simulink model "simulationBallCatching"  (R2017b)
settings: Solver=VariableStepAuto  StartTime=0.0  StopTime=simTime  MaxStep=0.001  RelTol=1e-3  EnableMultiTasking=on
undefined symbols (not defined in the file or in its folder): ball_radius, basket_side, contact_damping, contact_stiffness, dt, g, I11, I22, I33, Kd_phi, Kd_psi, Kd_theta, Kd_x, Kd_y, Kd_z, Kp_phi, Kp_psi, Kp_theta, Kp_x, Kp_y, Kp_z, m, m_ball, T, X, Y, Z, z0
libraries: nesl_utility x86, sm_lib x74, Contact_Forces_Lib x20, simulink x10
(part 3 of 4)

== system simulationBallCatching/Plant/Basket/Contact2 ==
  Bus Creator : BusCreator  Inputs=3
  Check Sphere on Plane : Subsystem
  Demux : Subsystem
  Enable Outputs : Subsystem
  External Force and Torque PlaB : sm_lib/Forces and Torques/External Force and Torque  ForceResolutionFrame=AttachedFrame  EnableForceX=off  EnableForceY=off  EnableForceZ=off  EnableForce=on  TorqueResolutionFrame=AttachedFrame  EnableTorqueX=off  EnableTorqueY=off  EnableTorqueZ=off  EnableTorque=on
  External Force and Torque SphF : sm_lib/Forces and Torques/External Force and Torque  ForceResolutionFrame=AttachedFrame  EnableForceX=off  EnableForceY=off  EnableForceZ=off  EnableForce=on  TorqueResolutionFrame=AttachedFrame  EnableTorqueX=off  EnableTorqueY=off  EnableTorqueZ=off  EnableTorque=on
  Forces : Subsystem
  If1 : If  IfExpression=u1>0
  Merge : Merge
  No Force : Subsystem  TreatAsAtomicUnit=on
  Sensing : Subsystem
  Transform nZ : sm_lib/Frames and Transforms/Rigid Transform  TranslationMethod=StandardAxis  TranslationStandardOffset=plane_depth-vis_len_plaBz/2  TranslationLengthUnit=m  TranslationStandardAxis=-Z  TranslationCartesianOffset=[0 0 0]  TranslationROffset=0  TranslationROffsetUnits=m  TranslationZOffset=0  TranslationZOffsetUnits=m  TranslationThetaOffset=0  TranslationThetaOffsetUnits=deg  RotationMethod=None  RotationAngleUnits=deg  RotationStandardAxis=+Z  RotationAngle=0.0  RotationArbitraryAxis=[0 0 1]  FollAlignAxisA=+X  BaseAlignAxisA=+Y  FollAlignAxisB=+Y  BaseAlignAxisB=+Z  RotationSequenceAxes=FollowerAxes  RotationSequence=XYX  RotationSequenceAngles=[0 0 0]  RotationSequenceAnglesUnits=deg  RotationMatrix=[1 0 0; 0 1 0; 0 0 1]
  Transform pZ : sm_lib/Frames and Transforms/Rigid Transform  TranslationMethod=StandardAxis  TranslationStandardOffset=plane_depth-vis_len_plaBz/2  TranslationLengthUnit=m  TranslationStandardAxis=+Z  TranslationCartesianOffset=[0 0 0]  TranslationROffset=0  TranslationROffsetUnits=m  TranslationZOffset=0  TranslationZOffsetUnits=m  TranslationThetaOffset=0  TranslationThetaOffsetUnits=deg  RotationMethod=None  RotationAngleUnits=deg  RotationStandardAxis=+Z  RotationAngle=0.0  RotationArbitraryAxis=[0 0 1]  FollAlignAxisA=+X  BaseAlignAxisA=+Y  FollAlignAxisB=+Y  BaseAlignAxisB=+Z  RotationSequenceAxes=FollowerAxes  RotationSequence=XYX  RotationSequenceAngles=[0 0 0]  RotationSequenceAnglesUnits=deg  RotationMatrix=[1 0 0; 0 1 0; 0 0 1]
  Visual CirF : sm_lib/Body Elements/Solid  InertiaType=CalculateFromGeometry  Mass=1  MassUnits=kg  CenterOfMass=[0 0 0]  CenterOfMassUnits=m  MomentsOfInertia=[1 1 1]  MomentsOfInertiaUnits=kg*m^2  ProductsOfInertia=[0 0 0]  ProductsOfInertiaUnits=kg*m^2  DensityBased=on  Density=0  DensityUnits=kg/(m^3)  DoExposeReferenceFrame=on  SerializedFrames=<Frames/>  GraphicType=FromGeometry  MarkerShape=Sphere  MarkerSize=10  GraphicVisPropType=SimpleVisualProperties  GraphicDiffuseColor=vis_clr  GraphicSpecularColor=[0.5 0.5 0.5 1.0]  GraphicAmbientColor=[0.15 0.15 0.15 1.0]  GraphicEmissiveColor=[0.0 0.0 0.0 1.0]  GraphicShininess=75  GraphicOpacity=vis_opc*vis_opc_en  GeometryShape=Sphere  RectangleSize=[1 1]  RectangleSizeUnits=m  BrickDimensions=[1 1 1]  BrickDimensionUnits=m  CylinderRadius=1  CylinderRadiusUnits=m  CylinderLength=1  CylinderLengthUnits=m  SphereRadius=sphere_rad  SphereRadiusUnits=m  EllipsoidRadii=[1 1 1]  EllipsoidRadiiUnits=m  ExtrusionCrossSection=[1 1; -1 1; -1 -1; 1 -1]  ExtrusionCrossSectionUnits=m  ExtrusionLength=1  ExtrusionLengthUnits=m  PolygonNumSides=3  PolygonOuterRadius=1  PolygonOuterRadiusUnits=m  ExtGeomFileType=STEP  ExtGeomFileUnits=m  RevolutionCrossSection=[1 1; 1 -1; 2 -1; 2 1]  RevolutionCrossSectionUnits=m  RevolutionExtent=Full  RevolutionAngle=180  RevolutionAngleUnits=deg
  Visual PlaBnZ : sm_lib/Body Elements/Solid  InertiaType=CalculateFromGeometry  Mass=1  MassUnits=kg  CenterOfMass=[0 0 0]  CenterOfMassUnits=m  MomentsOfInertia=[1 1 1]  MomentsOfInertiaUnits=kg*m^2  ProductsOfInertia=[0 0 0]  ProductsOfInertiaUnits=kg*m^2  DensityBased=on  Density=0  DensityUnits=kg/(m^3)  DoExposeReferenceFrame=on  SerializedFrames=<Frames/>  GraphicType=FromGeometry  MarkerShape=Sphere  MarkerSize=10  GraphicVisPropType=SimpleVisualProperties  GraphicDiffuseColor=vis_clr  GraphicSpecularColor=[0.5 0.5 0.5 1.0]  GraphicAmbientColor=[0.15 0.15 0.15 1.0]  GraphicEmissiveColor=[0.0 0.0 0.0 1.0]  GraphicShininess=75  GraphicOpacity=vis_opc*vis_opc_en  GeometryShape=Brick  RectangleSize=[1 1]  RectangleSizeUnits=m  BrickDimensions=[plane_lenx plane_leny vis_len_plaBz]  BrickDimensionUnits=m  CylinderRadius=1  CylinderRadiusUnits=m  CylinderLength=1  CylinderLengthUnits=m  SphereRadius=1  SphereRadiusUnits=m  EllipsoidRadii=[1 1 1]  EllipsoidRadiiUnits=m  ExtrusionCrossSection=[1 1; -1 1; -1 -1; 1 -1]  ExtrusionCrossSectionUnits=m  ExtrusionLength=1  ExtrusionLengthUnits=m  PolygonNumSides=3  PolygonOuterRadius=1  PolygonOuterRadiusUnits=m  ExtGeomFileType=STEP  ExtGeomFileUnits=m  RevolutionCrossSection=[1 1; 1 -1; 2 -1; 2 1]  RevolutionCrossSectionUnits=m  RevolutionExtent=Full  RevolutionAngle=180  RevolutionAngleUnits=deg
  Visual PlaBpZ : sm_lib/Body Elements/Solid  InertiaType=CalculateFromGeometry  Mass=1  MassUnits=kg  CenterOfMass=[0 0 0]  CenterOfMassUnits=m  MomentsOfInertia=[1 1 1]  MomentsOfInertiaUnits=kg*m^2  ProductsOfInertia=[0 0 0]  ProductsOfInertiaUnits=kg*m^2  DensityBased=on  Density=0  DensityUnits=kg/(m^3)  DoExposeReferenceFrame=on  SerializedFrames=<Frames/>  GraphicType=FromGeometry  MarkerShape=Sphere  MarkerSize=10  GraphicVisPropType=SimpleVisualProperties  GraphicDiffuseColor=vis_clr  GraphicSpecularColor=[0.5 0.5 0.5 1.0]  GraphicAmbientColor=[0.15 0.15 0.15 1.0]  GraphicEmissiveColor=[0.0 0.0 0.0 1.0]  GraphicShininess=75  GraphicOpacity=vis_opc*vis_opc_en  GeometryShape=Brick  RectangleSize=[1 1]  RectangleSizeUnits=m  BrickDimensions=[plane_lenx plane_leny vis_len_plaBz]  BrickDimensionUnits=m  CylinderRadius=1  CylinderRadiusUnits=m  CylinderLength=1  CylinderLengthUnits=m  SphereRadius=1  SphereRadiusUnits=m  EllipsoidRadii=[1 1 1]  EllipsoidRadiiUnits=m  ExtrusionCrossSection=[1 1; -1 1; -1 -1; 1 -1]  ExtrusionCrossSectionUnits=m  ExtrusionLength=1  ExtrusionLengthUnits=m  PolygonNumSides=3  PolygonOuterRadius=1  PolygonOuterRadiusUnits=m  ExtGeomFileType=STEP  ExtGeomFileUnits=m  RevolutionCrossSection=[1 1; 1 -1; 2 -1; 2 1]  RevolutionCrossSectionUnits=m  RevolutionExtent=Full  RevolutionAngle=180  RevolutionAngleUnits=deg
  SphF : PMIOPort  Port=1  Side=Left
  PlaB : PMIOPort  Port=2  Side=Right
  Out : Outport
  wires:
  Check Sphere on Plane/1(En) -> If1/1, Enable Outputs/2(En)
  Enable Outputs/1(Out) -> Out/1
  Bus Creator/1 -> Enable Outputs/3(FrameSep)  "Frame Sep"
  Forces/2(Out) -> Enable Outputs/1(Frc)
  Merge/1 -> Demux/1(Frc)  "FSph"
  Forces/1(Frc) -> Merge/2
  Sensing/4(vz) -> Forces/4(vz)
  Sensing/5(R) -> Forces/5(R)
  Sensing/3(z) -> Forces/3(z), Bus Creator/3  "z"
  Sensing/6(wx) -> Forces/6(wx)
  Sensing/7(wy) -> Forces/7(wy)
  Sensing/8(vx) -> Forces/8(vx)
  Sensing/9(vy) -> Forces/9(vy)
  Sensing/1(x) -> Forces/1(x), Bus Creator/1, Check Sphere on Plane/1(x)  "x"
  Sensing/2(y) -> Forces/2(y), Bus Creator/2, Check Sphere on Plane/2(y)  "y"
  If1/1 -> Forces/Action
  If1/2 -> No Force/Action
  No Force/1(Frc) -> Merge/1
  connections:
  SphF/RConn1 -- Sensing/LConn1 -- Visual CirF/RConn1 -- External Force and Torque SphF/RConn1
  PlaB/RConn1 -- Sensing/LConn2 -- External Force and Torque PlaB/RConn1 -- Transform pZ/LConn1 -- Transform nZ/LConn1
  Demux/RConn1 -- External Force and Torque SphF/LConn1
  Demux/RConn2 -- External Force and Torque SphF/LConn2
  Demux/RConn3 -- External Force and Torque PlaB/LConn1
  Demux/RConn4 -- External Force and Torque PlaB/LConn2
  Transform pZ/RConn1 -- Visual PlaBpZ/RConn1
  Transform nZ/RConn1 -- Visual PlaBnZ/RConn1

== system simulationBallCatching/Plant/Basket/Contact3 ==
  Bus Creator : BusCreator  Inputs=3
  Check Sphere on Plane : Subsystem
  Demux : Subsystem
  Enable Outputs : Subsystem
  External Force and Torque PlaB : sm_lib/Forces and Torques/External Force and Torque  ForceResolutionFrame=AttachedFrame  EnableForceX=off  EnableForceY=off  EnableForceZ=off  EnableForce=on  TorqueResolutionFrame=AttachedFrame  EnableTorqueX=off  EnableTorqueY=off  EnableTorqueZ=off  EnableTorque=on
  External Force and Torque SphF : sm_lib/Forces and Torques/External Force and Torque  ForceResolutionFrame=AttachedFrame  EnableForceX=off  EnableForceY=off  EnableForceZ=off  EnableForce=on  TorqueResolutionFrame=AttachedFrame  EnableTorqueX=off  EnableTorqueY=off  EnableTorqueZ=off  EnableTorque=on
  Forces : Subsystem
  If1 : If  IfExpression=u1>0
  Merge : Merge
  No Force : Subsystem  TreatAsAtomicUnit=on
  Sensing : Subsystem
  Transform nZ : sm_lib/Frames and Transforms/Rigid Transform  TranslationMethod=StandardAxis  TranslationStandardOffset=plane_depth-vis_len_plaBz/2  TranslationLengthUnit=m  TranslationStandardAxis=-Z  TranslationCartesianOffset=[0 0 0]  TranslationROffset=0  TranslationROffsetUnits=m  TranslationZOffset=0  TranslationZOffsetUnits=m  TranslationThetaOffset=0  TranslationThetaOffsetUnits=deg  RotationMethod=None  RotationAngleUnits=deg  RotationStandardAxis=+Z  RotationAngle=0.0  RotationArbitraryAxis=[0 0 1]  FollAlignAxisA=+X  BaseAlignAxisA=+Y  FollAlignAxisB=+Y  BaseAlignAxisB=+Z  RotationSequenceAxes=FollowerAxes  RotationSequence=XYX  RotationSequenceAngles=[0 0 0]  RotationSequenceAnglesUnits=deg  RotationMatrix=[1 0 0; 0 1 0; 0 0 1]
  Transform pZ : sm_lib/Frames and Transforms/Rigid Transform  TranslationMethod=StandardAxis  TranslationStandardOffset=plane_depth-vis_len_plaBz/2  TranslationLengthUnit=m  TranslationStandardAxis=+Z  TranslationCartesianOffset=[0 0 0]  TranslationROffset=0  TranslationROffsetUnits=m  TranslationZOffset=0  TranslationZOffsetUnits=m  TranslationThetaOffset=0  TranslationThetaOffsetUnits=deg  RotationMethod=None  RotationAngleUnits=deg  RotationStandardAxis=+Z  RotationAngle=0.0  RotationArbitraryAxis=[0 0 1]  FollAlignAxisA=+X  BaseAlignAxisA=+Y  FollAlignAxisB=+Y  BaseAlignAxisB=+Z  RotationSequenceAxes=FollowerAxes  RotationSequence=XYX  RotationSequenceAngles=[0 0 0]  RotationSequenceAnglesUnits=deg  RotationMatrix=[1 0 0; 0 1 0; 0 0 1]
  Visual CirF : sm_lib/Body Elements/Solid  InertiaType=CalculateFromGeometry  Mass=1  MassUnits=kg  CenterOfMass=[0 0 0]  CenterOfMassUnits=m  MomentsOfInertia=[1 1 1]  MomentsOfInertiaUnits=kg*m^2  ProductsOfInertia=[0 0 0]  ProductsOfInertiaUnits=kg*m^2  DensityBased=on  Density=0  DensityUnits=kg/(m^3)  DoExposeReferenceFrame=on  SerializedFrames=<Frames/>  GraphicType=FromGeometry  MarkerShape=Sphere  MarkerSize=10  GraphicVisPropType=SimpleVisualProperties  GraphicDiffuseColor=vis_clr  GraphicSpecularColor=[0.5 0.5 0.5 1.0]  GraphicAmbientColor=[0.15 0.15 0.15 1.0]  GraphicEmissiveColor=[0.0 0.0 0.0 1.0]  GraphicShininess=75  GraphicOpacity=vis_opc*vis_opc_en  GeometryShape=Sphere  RectangleSize=[1 1]  RectangleSizeUnits=m  BrickDimensions=[1 1 1]  BrickDimensionUnits=m  CylinderRadius=1  CylinderRadiusUnits=m  CylinderLength=1  CylinderLengthUnits=m  SphereRadius=sphere_rad  SphereRadiusUnits=m  EllipsoidRadii=[1 1 1]  EllipsoidRadiiUnits=m  ExtrusionCrossSection=[1 1; -1 1; -1 -1; 1 -1]  ExtrusionCrossSectionUnits=m  ExtrusionLength=1  ExtrusionLengthUnits=m  PolygonNumSides=3  PolygonOuterRadius=1  PolygonOuterRadiusUnits=m  ExtGeomFileType=STEP  ExtGeomFileUnits=m  RevolutionCrossSection=[1 1; 1 -1; 2 -1; 2 1]  RevolutionCrossSectionUnits=m  RevolutionExtent=Full  RevolutionAngle=180  RevolutionAngleUnits=deg
  Visual PlaBnZ : sm_lib/Body Elements/Solid  InertiaType=CalculateFromGeometry  Mass=1  MassUnits=kg  CenterOfMass=[0 0 0]  CenterOfMassUnits=m  MomentsOfInertia=[1 1 1]  MomentsOfInertiaUnits=kg*m^2  ProductsOfInertia=[0 0 0]  ProductsOfInertiaUnits=kg*m^2  DensityBased=on  Density=0  DensityUnits=kg/(m^3)  DoExposeReferenceFrame=on  SerializedFrames=<Frames/>  GraphicType=FromGeometry  MarkerShape=Sphere  MarkerSize=10  GraphicVisPropType=SimpleVisualProperties  GraphicDiffuseColor=vis_clr  GraphicSpecularColor=[0.5 0.5 0.5 1.0]  GraphicAmbientColor=[0.15 0.15 0.15 1.0]  GraphicEmissiveColor=[0.0 0.0 0.0 1.0]  GraphicShininess=75  GraphicOpacity=vis_opc*vis_opc_en  GeometryShape=Brick  RectangleSize=[1 1]  RectangleSizeUnits=m  BrickDimensions=[plane_lenx plane_leny vis_len_plaBz]  BrickDimensionUnits=m  CylinderRadius=1  CylinderRadiusUnits=m  CylinderLength=1  CylinderLengthUnits=m  SphereRadius=1  SphereRadiusUnits=m  EllipsoidRadii=[1 1 1]  EllipsoidRadiiUnits=m  ExtrusionCrossSection=[1 1; -1 1; -1 -1; 1 -1]  ExtrusionCrossSectionUnits=m  ExtrusionLength=1  ExtrusionLengthUnits=m  PolygonNumSides=3  PolygonOuterRadius=1  PolygonOuterRadiusUnits=m  ExtGeomFileType=STEP  ExtGeomFileUnits=m  RevolutionCrossSection=[1 1; 1 -1; 2 -1; 2 1]  RevolutionCrossSectionUnits=m  RevolutionExtent=Full  RevolutionAngle=180  RevolutionAngleUnits=deg
  Visual PlaBpZ : sm_lib/Body Elements/Solid  InertiaType=CalculateFromGeometry  Mass=1  MassUnits=kg  CenterOfMass=[0 0 0]  CenterOfMassUnits=m  MomentsOfInertia=[1 1 1]  MomentsOfInertiaUnits=kg*m^2  ProductsOfInertia=[0 0 0]  ProductsOfInertiaUnits=kg*m^2  DensityBased=on  Density=0  DensityUnits=kg/(m^3)  DoExposeReferenceFrame=on  SerializedFrames=<Frames/>  GraphicType=FromGeometry  MarkerShape=Sphere  MarkerSize=10  GraphicVisPropType=SimpleVisualProperties  GraphicDiffuseColor=vis_clr  GraphicSpecularColor=[0.5 0.5 0.5 1.0]  GraphicAmbientColor=[0.15 0.15 0.15 1.0]  GraphicEmissiveColor=[0.0 0.0 0.0 1.0]  GraphicShininess=75  GraphicOpacity=vis_opc*vis_opc_en  GeometryShape=Brick  RectangleSize=[1 1]  RectangleSizeUnits=m  BrickDimensions=[plane_lenx plane_leny vis_len_plaBz]  BrickDimensionUnits=m  CylinderRadius=1  CylinderRadiusUnits=m  CylinderLength=1  CylinderLengthUnits=m  SphereRadius=1  SphereRadiusUnits=m  EllipsoidRadii=[1 1 1]  EllipsoidRadiiUnits=m  ExtrusionCrossSection=[1 1; -1 1; -1 -1; 1 -1]  ExtrusionCrossSectionUnits=m  ExtrusionLength=1  ExtrusionLengthUnits=m  PolygonNumSides=3  PolygonOuterRadius=1  PolygonOuterRadiusUnits=m  ExtGeomFileType=STEP  ExtGeomFileUnits=m  RevolutionCrossSection=[1 1; 1 -1; 2 -1; 2 1]  RevolutionCrossSectionUnits=m  RevolutionExtent=Full  RevolutionAngle=180  RevolutionAngleUnits=deg
  SphF : PMIOPort  Port=1  Side=Left
  PlaB : PMIOPort  Port=2  Side=Right
  Out : Outport
  wires:
  Check Sphere on Plane/1(En) -> If1/1, Enable Outputs/2(En)
  Enable Outputs/1(Out) -> Out/1
  Bus Creator/1 -> Enable Outputs/3(FrameSep)  "Frame Sep"
  Forces/2(Out) -> Enable Outputs/1(Frc)
  Merge/1 -> Demux/1(Frc)  "FSph"
  Forces/1(Frc) -> Merge/2
  Sensing/4(vz) -> Forces/4(vz)
  Sensing/5(R) -> Forces/5(R)
  Sensing/3(z) -> Forces/3(z), Bus Creator/3  "z"
  Sensing/6(wx) -> Forces/6(wx)
  Sensing/7(wy) -> Forces/7(wy)
  Sensing/8(vx) -> Forces/8(vx)
  Sensing/9(vy) -> Forces/9(vy)
  Sensing/1(x) -> Forces/1(x), Bus Creator/1, Check Sphere on Plane/1(x)  "x"
  Sensing/2(y) -> Forces/2(y), Bus Creator/2, Check Sphere on Plane/2(y)  "y"
  If1/1 -> Forces/Action
  If1/2 -> No Force/Action
  No Force/1(Frc) -> Merge/1
  connections:
  SphF/RConn1 -- Sensing/LConn1 -- Visual CirF/RConn1 -- External Force and Torque SphF/RConn1
  PlaB/RConn1 -- Sensing/LConn2 -- External Force and Torque PlaB/RConn1 -- Transform pZ/LConn1 -- Transform nZ/LConn1
  Demux/RConn1 -- External Force and Torque SphF/LConn1
  Demux/RConn2 -- External Force and Torque SphF/LConn2
  Demux/RConn3 -- External Force and Torque PlaB/LConn1
  Demux/RConn4 -- External Force and Torque PlaB/LConn2
  Transform pZ/RConn1 -- Visual PlaBpZ/RConn1
  Transform nZ/RConn1 -- Visual PlaBnZ/RConn1

== system simulationBallCatching/Plant/Basket/Contact4 ==
  Bus Creator : BusCreator  Inputs=3
  Check Sphere on Plane : Subsystem
  Demux : Subsystem
  Enable Outputs : Subsystem
  External Force and Torque PlaB : sm_lib/Forces and Torques/External Force and Torque  ForceResolutionFrame=AttachedFrame  EnableForceX=off  EnableForceY=off  EnableForceZ=off  EnableForce=on  TorqueResolutionFrame=AttachedFrame  EnableTorqueX=off  EnableTorqueY=off  EnableTorqueZ=off  EnableTorque=on
  External Force and Torque SphF : sm_lib/Forces and Torques/External Force and Torque  ForceResolutionFrame=AttachedFrame  EnableForceX=off  EnableForceY=off  EnableForceZ=off  EnableForce=on  TorqueResolutionFrame=AttachedFrame  EnableTorqueX=off  EnableTorqueY=off  EnableTorqueZ=off  EnableTorque=on
  Forces : Subsystem
  If1 : If  IfExpression=u1>0
  Merge : Merge
  No Force : Subsystem  TreatAsAtomicUnit=on
  Sensing : Subsystem
  Transform nZ : sm_lib/Frames and Transforms/Rigid Transform  TranslationMethod=StandardAxis  TranslationStandardOffset=plane_depth-vis_len_plaBz/2  TranslationLengthUnit=m  TranslationStandardAxis=-Z  TranslationCartesianOffset=[0 0 0]  TranslationROffset=0  TranslationROffsetUnits=m  TranslationZOffset=0  TranslationZOffsetUnits=m  TranslationThetaOffset=0  TranslationThetaOffsetUnits=deg  RotationMethod=None  RotationAngleUnits=deg  RotationStandardAxis=+Z  RotationAngle=0.0  RotationArbitraryAxis=[0 0 1]  FollAlignAxisA=+X  BaseAlignAxisA=+Y  FollAlignAxisB=+Y  BaseAlignAxisB=+Z  RotationSequenceAxes=FollowerAxes  RotationSequence=XYX  RotationSequenceAngles=[0 0 0]  RotationSequenceAnglesUnits=deg  RotationMatrix=[1 0 0; 0 1 0; 0 0 1]
  Transform pZ : sm_lib/Frames and Transforms/Rigid Transform  TranslationMethod=StandardAxis  TranslationStandardOffset=plane_depth-vis_len_plaBz/2  TranslationLengthUnit=m  TranslationStandardAxis=+Z  TranslationCartesianOffset=[0 0 0]  TranslationROffset=0  TranslationROffsetUnits=m  TranslationZOffset=0  TranslationZOffsetUnits=m  TranslationThetaOffset=0  TranslationThetaOffsetUnits=deg  RotationMethod=None  RotationAngleUnits=deg  RotationStandardAxis=+Z  RotationAngle=0.0  RotationArbitraryAxis=[0 0 1]  FollAlignAxisA=+X  BaseAlignAxisA=+Y  FollAlignAxisB=+Y  BaseAlignAxisB=+Z  RotationSequenceAxes=FollowerAxes  RotationSequence=XYX  RotationSequenceAngles=[0 0 0]  RotationSequenceAnglesUnits=deg  RotationMatrix=[1 0 0; 0 1 0; 0 0 1]
  Visual CirF : sm_lib/Body Elements/Solid  InertiaType=CalculateFromGeometry  Mass=1  MassUnits=kg  CenterOfMass=[0 0 0]  CenterOfMassUnits=m  MomentsOfInertia=[1 1 1]  MomentsOfInertiaUnits=kg*m^2  ProductsOfInertia=[0 0 0]  ProductsOfInertiaUnits=kg*m^2  DensityBased=on  Density=0  DensityUnits=kg/(m^3)  DoExposeReferenceFrame=on  SerializedFrames=<Frames/>  GraphicType=FromGeometry  MarkerShape=Sphere  MarkerSize=10  GraphicVisPropType=SimpleVisualProperties  GraphicDiffuseColor=vis_clr  GraphicSpecularColor=[0.5 0.5 0.5 1.0]  GraphicAmbientColor=[0.15 0.15 0.15 1.0]  GraphicEmissiveColor=[0.0 0.0 0.0 1.0]  GraphicShininess=75  GraphicOpacity=vis_opc*vis_opc_en  GeometryShape=Sphere  RectangleSize=[1 1]  RectangleSizeUnits=m  BrickDimensions=[1 1 1]  BrickDimensionUnits=m  CylinderRadius=1  CylinderRadiusUnits=m  CylinderLength=1  CylinderLengthUnits=m  SphereRadius=sphere_rad  SphereRadiusUnits=m  EllipsoidRadii=[1 1 1]  EllipsoidRadiiUnits=m  ExtrusionCrossSection=[1 1; -1 1; -1 -1; 1 -1]  ExtrusionCrossSectionUnits=m  ExtrusionLength=1  ExtrusionLengthUnits=m  PolygonNumSides=3  PolygonOuterRadius=1  PolygonOuterRadiusUnits=m  ExtGeomFileType=STEP  ExtGeomFileUnits=m  RevolutionCrossSection=[1 1; 1 -1; 2 -1; 2 1]  RevolutionCrossSectionUnits=m  RevolutionExtent=Full  RevolutionAngle=180  RevolutionAngleUnits=deg
  Visual PlaBnZ : sm_lib/Body Elements/Solid  InertiaType=CalculateFromGeometry  Mass=1  MassUnits=kg  CenterOfMass=[0 0 0]  CenterOfMassUnits=m  MomentsOfInertia=[1 1 1]  MomentsOfInertiaUnits=kg*m^2  ProductsOfInertia=[0 0 0]  ProductsOfInertiaUnits=kg*m^2  DensityBased=on  Density=0  DensityUnits=kg/(m^3)  DoExposeReferenceFrame=on  SerializedFrames=<Frames/>  GraphicType=FromGeometry  MarkerShape=Sphere  MarkerSize=10  GraphicVisPropType=SimpleVisualProperties  GraphicDiffuseColor=vis_clr  GraphicSpecularColor=[0.5 0.5 0.5 1.0]  GraphicAmbientColor=[0.15 0.15 0.15 1.0]  GraphicEmissiveColor=[0.0 0.0 0.0 1.0]  GraphicShininess=75  GraphicOpacity=vis_opc*vis_opc_en  GeometryShape=Brick  RectangleSize=[1 1]  RectangleSizeUnits=m  BrickDimensions=[plane_lenx plane_leny vis_len_plaBz]  BrickDimensionUnits=m  CylinderRadius=1  CylinderRadiusUnits=m  CylinderLength=1  CylinderLengthUnits=m  SphereRadius=1  SphereRadiusUnits=m  EllipsoidRadii=[1 1 1]  EllipsoidRadiiUnits=m  ExtrusionCrossSection=[1 1; -1 1; -1 -1; 1 -1]  ExtrusionCrossSectionUnits=m  ExtrusionLength=1  ExtrusionLengthUnits=m  PolygonNumSides=3  PolygonOuterRadius=1  PolygonOuterRadiusUnits=m  ExtGeomFileType=STEP  ExtGeomFileUnits=m  RevolutionCrossSection=[1 1; 1 -1; 2 -1; 2 1]  RevolutionCrossSectionUnits=m  RevolutionExtent=Full  RevolutionAngle=180  RevolutionAngleUnits=deg
  Visual PlaBpZ : sm_lib/Body Elements/Solid  InertiaType=CalculateFromGeometry  Mass=1  MassUnits=kg  CenterOfMass=[0 0 0]  CenterOfMassUnits=m  MomentsOfInertia=[1 1 1]  MomentsOfInertiaUnits=kg*m^2  ProductsOfInertia=[0 0 0]  ProductsOfInertiaUnits=kg*m^2  DensityBased=on  Density=0  DensityUnits=kg/(m^3)  DoExposeReferenceFrame=on  SerializedFrames=<Frames/>  GraphicType=FromGeometry  MarkerShape=Sphere  MarkerSize=10  GraphicVisPropType=SimpleVisualProperties  GraphicDiffuseColor=vis_clr  GraphicSpecularColor=[0.5 0.5 0.5 1.0]  GraphicAmbientColor=[0.15 0.15 0.15 1.0]  GraphicEmissiveColor=[0.0 0.0 0.0 1.0]  GraphicShininess=75  GraphicOpacity=vis_opc*vis_opc_en  GeometryShape=Brick  RectangleSize=[1 1]  RectangleSizeUnits=m  BrickDimensions=[plane_lenx plane_leny vis_len_plaBz]  BrickDimensionUnits=m  CylinderRadius=1  CylinderRadiusUnits=m  CylinderLength=1  CylinderLengthUnits=m  SphereRadius=1  SphereRadiusUnits=m  EllipsoidRadii=[1 1 1]  EllipsoidRadiiUnits=m  ExtrusionCrossSection=[1 1; -1 1; -1 -1; 1 -1]  ExtrusionCrossSectionUnits=m  ExtrusionLength=1  ExtrusionLengthUnits=m  PolygonNumSides=3  PolygonOuterRadius=1  PolygonOuterRadiusUnits=m  ExtGeomFileType=STEP  ExtGeomFileUnits=m  RevolutionCrossSection=[1 1; 1 -1; 2 -1; 2 1]  RevolutionCrossSectionUnits=m  RevolutionExtent=Full  RevolutionAngle=180  RevolutionAngleUnits=deg
  SphF : PMIOPort  Port=1  Side=Left
  PlaB : PMIOPort  Port=2  Side=Right
  Out : Outport
  wires:
  Check Sphere on Plane/1(En) -> If1/1, Enable Outputs/2(En)
  Enable Outputs/1(Out) -> Out/1
  Bus Creator/1 -> Enable Outputs/3(FrameSep)  "Frame Sep"
  Forces/2(Out) -> Enable Outputs/1(Frc)
  Merge/1 -> Demux/1(Frc)  "FSph"
  Forces/1(Frc) -> Merge/2
  Sensing/4(vz) -> Forces/4(vz)
  Sensing/5(R) -> Forces/5(R)
  Sensing/3(z) -> Forces/3(z), Bus Creator/3  "z"
  Sensing/6(wx) -> Forces/6(wx)
  Sensing/7(wy) -> Forces/7(wy)
  Sensing/8(vx) -> Forces/8(vx)
  Sensing/9(vy) -> Forces/9(vy)
  Sensing/1(x) -> Forces/1(x), Bus Creator/1, Check Sphere on Plane/1(x)  "x"
  Sensing/2(y) -> Forces/2(y), Bus Creator/2, Check Sphere on Plane/2(y)  "y"
  If1/1 -> Forces/Action
  If1/2 -> No Force/Action
  No Force/1(Frc) -> Merge/1
  connections:
  SphF/RConn1 -- Sensing/LConn1 -- Visual CirF/RConn1 -- External Force and Torque SphF/RConn1
  PlaB/RConn1 -- Sensing/LConn2 -- External Force and Torque PlaB/RConn1 -- Transform pZ/LConn1 -- Transform nZ/LConn1
  Demux/RConn1 -- External Force and Torque SphF/LConn1
  Demux/RConn2 -- External Force and Torque SphF/LConn2
  Demux/RConn3 -- External Force and Torque PlaB/LConn1
  Demux/RConn4 -- External Force and Torque PlaB/LConn2
  Transform pZ/RConn1 -- Visual PlaBpZ/RConn1
  Transform nZ/RConn1 -- Visual PlaBnZ/RConn1

== system simulationBallCatching/Plant/Basket/Contact6 ==
  Bus Creator : BusCreator  Inputs=3
  Check Sphere on Plane : Subsystem
  Demux : Subsystem
  Enable Outputs : Subsystem
  External Force and Torque PlaB : sm_lib/Forces and Torques/External Force and Torque  ForceResolutionFrame=AttachedFrame  EnableForceX=off  EnableForceY=off  EnableForceZ=off  EnableForce=on  TorqueResolutionFrame=AttachedFrame  EnableTorqueX=off  EnableTorqueY=off  EnableTorqueZ=off  EnableTorque=on
  External Force and Torque SphF : sm_lib/Forces and Torques/External Force and Torque  ForceResolutionFrame=AttachedFrame  EnableForceX=off  EnableForceY=off  EnableForceZ=off  EnableForce=on  TorqueResolutionFrame=AttachedFrame  EnableTorqueX=off  EnableTorqueY=off  EnableTorqueZ=off  EnableTorque=on
  Forces : Subsystem
  If1 : If  IfExpression=u1>0
  Merge : Merge
  No Force : Subsystem  TreatAsAtomicUnit=on
  Sensing : Subsystem
  Transform nZ : sm_lib/Frames and Transforms/Rigid Transform  TranslationMethod=StandardAxis  TranslationStandardOffset=plane_depth-vis_len_plaBz/2  TranslationLengthUnit=m  TranslationStandardAxis=-Z  TranslationCartesianOffset=[0 0 0]  TranslationROffset=0  TranslationROffsetUnits=m  TranslationZOffset=0  TranslationZOffsetUnits=m  TranslationThetaOffset=0  TranslationThetaOffsetUnits=deg  RotationMethod=None  RotationAngleUnits=deg  RotationStandardAxis=+Z  RotationAngle=0.0  RotationArbitraryAxis=[0 0 1]  FollAlignAxisA=+X  BaseAlignAxisA=+Y  FollAlignAxisB=+Y  BaseAlignAxisB=+Z  RotationSequenceAxes=FollowerAxes  RotationSequence=XYX  RotationSequenceAngles=[0 0 0]  RotationSequenceAnglesUnits=deg  RotationMatrix=[1 0 0; 0 1 0; 0 0 1]
  Transform pZ : sm_lib/Frames and Transforms/Rigid Transform  TranslationMethod=StandardAxis  TranslationStandardOffset=plane_depth-vis_len_plaBz/2  TranslationLengthUnit=m  TranslationStandardAxis=+Z  TranslationCartesianOffset=[0 0 0]  TranslationROffset=0  TranslationROffsetUnits=m  TranslationZOffset=0  TranslationZOffsetUnits=m  TranslationThetaOffset=0  TranslationThetaOffsetUnits=deg  RotationMethod=None  RotationAngleUnits=deg  RotationStandardAxis=+Z  RotationAngle=0.0  RotationArbitraryAxis=[0 0 1]  FollAlignAxisA=+X  BaseAlignAxisA=+Y  FollAlignAxisB=+Y  BaseAlignAxisB=+Z  RotationSequenceAxes=FollowerAxes  RotationSequence=XYX  RotationSequenceAngles=[0 0 0]  RotationSequenceAnglesUnits=deg  RotationMatrix=[1 0 0; 0 1 0; 0 0 1]
  Visual CirF : sm_lib/Body Elements/Solid  InertiaType=CalculateFromGeometry  Mass=1  MassUnits=kg  CenterOfMass=[0 0 0]  CenterOfMassUnits=m  MomentsOfInertia=[1 1 1]  MomentsOfInertiaUnits=kg*m^2  ProductsOfInertia=[0 0 0]  ProductsOfInertiaUnits=kg*m^2  DensityBased=on  Density=0  DensityUnits=kg/(m^3)  DoExposeReferenceFrame=on  SerializedFrames=<Frames/>  GraphicType=FromGeometry  MarkerShape=Sphere  MarkerSize=10  GraphicVisPropType=SimpleVisualProperties  GraphicDiffuseColor=vis_clr  GraphicSpecularColor=[0.5 0.5 0.5 1.0]  GraphicAmbientColor=[0.15 0.15 0.15 1.0]  GraphicEmissiveColor=[0.0 0.0 0.0 1.0]  GraphicShininess=75  GraphicOpacity=vis_opc*vis_opc_en  GeometryShape=Sphere  RectangleSize=[1 1]  RectangleSizeUnits=m  BrickDimensions=[1 1 1]  BrickDimensionUnits=m  CylinderRadius=1  CylinderRadiusUnits=m  CylinderLength=1  CylinderLengthUnits=m  SphereRadius=sphere_rad  SphereRadiusUnits=m  EllipsoidRadii=[1 1 1]  EllipsoidRadiiUnits=m  ExtrusionCrossSection=[1 1; -1 1; -1 -1; 1 -1]  ExtrusionCrossSectionUnits=m  ExtrusionLength=1  ExtrusionLengthUnits=m  PolygonNumSides=3  PolygonOuterRadius=1  PolygonOuterRadiusUnits=m  ExtGeomFileType=STEP  ExtGeomFileUnits=m  RevolutionCrossSection=[1 1; 1 -1; 2 -1; 2 1]  RevolutionCrossSectionUnits=m  RevolutionExtent=Full  RevolutionAngle=180  RevolutionAngleUnits=deg
  Visual PlaBnZ : sm_lib/Body Elements/Solid  InertiaType=CalculateFromGeometry  Mass=1  MassUnits=kg  CenterOfMass=[0 0 0]  CenterOfMassUnits=m  MomentsOfInertia=[1 1 1]  MomentsOfInertiaUnits=kg*m^2  ProductsOfInertia=[0 0 0]  ProductsOfInertiaUnits=kg*m^2  DensityBased=on  Density=0  DensityUnits=kg/(m^3)  DoExposeReferenceFrame=on  SerializedFrames=<Frames/>  GraphicType=FromGeometry  MarkerShape=Sphere  MarkerSize=10  GraphicVisPropType=SimpleVisualProperties  GraphicDiffuseColor=vis_clr  GraphicSpecularColor=[0.5 0.5 0.5 1.0]  GraphicAmbientColor=[0.15 0.15 0.15 1.0]  GraphicEmissiveColor=[0.0 0.0 0.0 1.0]  GraphicShininess=75  GraphicOpacity=vis_opc*vis_opc_en  GeometryShape=Brick  RectangleSize=[1 1]  RectangleSizeUnits=m  BrickDimensions=[plane_lenx plane_leny vis_len_plaBz]  BrickDimensionUnits=m  CylinderRadius=1  CylinderRadiusUnits=m  CylinderLength=1  CylinderLengthUnits=m  SphereRadius=1  SphereRadiusUnits=m  EllipsoidRadii=[1 1 1]  EllipsoidRadiiUnits=m  ExtrusionCrossSection=[1 1; -1 1; -1 -1; 1 -1]  ExtrusionCrossSectionUnits=m  ExtrusionLength=1  ExtrusionLengthUnits=m  PolygonNumSides=3  PolygonOuterRadius=1  PolygonOuterRadiusUnits=m  ExtGeomFileType=STEP  ExtGeomFileUnits=m  RevolutionCrossSection=[1 1; 1 -1; 2 -1; 2 1]  RevolutionCrossSectionUnits=m  RevolutionExtent=Full  RevolutionAngle=180  RevolutionAngleUnits=deg
  Visual PlaBpZ : sm_lib/Body Elements/Solid  InertiaType=CalculateFromGeometry  Mass=1  MassUnits=kg  CenterOfMass=[0 0 0]  CenterOfMassUnits=m  MomentsOfInertia=[1 1 1]  MomentsOfInertiaUnits=kg*m^2  ProductsOfInertia=[0 0 0]  ProductsOfInertiaUnits=kg*m^2  DensityBased=on  Density=0  DensityUnits=kg/(m^3)  DoExposeReferenceFrame=on  SerializedFrames=<Frames/>  GraphicType=FromGeometry  MarkerShape=Sphere  MarkerSize=10  GraphicVisPropType=SimpleVisualProperties  GraphicDiffuseColor=vis_clr  GraphicSpecularColor=[0.5 0.5 0.5 1.0]  GraphicAmbientColor=[0.15 0.15 0.15 1.0]  GraphicEmissiveColor=[0.0 0.0 0.0 1.0]  GraphicShininess=75  GraphicOpacity=vis_opc*vis_opc_en  GeometryShape=Brick  RectangleSize=[1 1]  RectangleSizeUnits=m  BrickDimensions=[plane_lenx plane_leny vis_len_plaBz]  BrickDimensionUnits=m  CylinderRadius=1  CylinderRadiusUnits=m  CylinderLength=1  CylinderLengthUnits=m  SphereRadius=1  SphereRadiusUnits=m  EllipsoidRadii=[1 1 1]  EllipsoidRadiiUnits=m  ExtrusionCrossSection=[1 1; -1 1; -1 -1; 1 -1]  ExtrusionCrossSectionUnits=m  ExtrusionLength=1  ExtrusionLengthUnits=m  PolygonNumSides=3  PolygonOuterRadius=1  PolygonOuterRadiusUnits=m  ExtGeomFileType=STEP  ExtGeomFileUnits=m  RevolutionCrossSection=[1 1; 1 -1; 2 -1; 2 1]  RevolutionCrossSectionUnits=m  RevolutionExtent=Full  RevolutionAngle=180  RevolutionAngleUnits=deg
  SphF : PMIOPort  Port=1  Side=Left
  PlaB : PMIOPort  Port=2  Side=Right
  Out : Outport
  wires:
  Check Sphere on Plane/1(En) -> If1/1, Enable Outputs/2(En)
  Enable Outputs/1(Out) -> Out/1
  Bus Creator/1 -> Enable Outputs/3(FrameSep)  "Frame Sep"
  Forces/2(Out) -> Enable Outputs/1(Frc)
  Merge/1 -> Demux/1(Frc)  "FSph"
  Forces/1(Frc) -> Merge/2
  Sensing/4(vz) -> Forces/4(vz)
  Sensing/5(R) -> Forces/5(R)
  Sensing/3(z) -> Forces/3(z), Bus Creator/3  "z"
  Sensing/6(wx) -> Forces/6(wx)
  Sensing/7(wy) -> Forces/7(wy)
  Sensing/8(vx) -> Forces/8(vx)
  Sensing/9(vy) -> Forces/9(vy)
  Sensing/1(x) -> Forces/1(x), Bus Creator/1, Check Sphere on Plane/1(x)  "x"
  Sensing/2(y) -> Forces/2(y), Bus Creator/2, Check Sphere on Plane/2(y)  "y"
  If1/1 -> Forces/Action
  If1/2 -> No Force/Action
  No Force/1(Frc) -> Merge/1
  connections:
  SphF/RConn1 -- Sensing/LConn1 -- Visual CirF/RConn1 -- External Force and Torque SphF/RConn1
  PlaB/RConn1 -- Sensing/LConn2 -- External Force and Torque PlaB/RConn1 -- Transform pZ/LConn1 -- Transform nZ/LConn1
  Demux/RConn1 -- External Force and Torque SphF/LConn1
  Demux/RConn2 -- External Force and Torque SphF/LConn2
  Demux/RConn3 -- External Force and Torque PlaB/LConn1
  Demux/RConn4 -- External Force and Torque PlaB/LConn2
  Transform pZ/RConn1 -- Visual PlaBpZ/RConn1
  Transform nZ/RConn1 -- Visual PlaBnZ/RConn1

== system simulationBallCatching/Plant/Basket/Contact1/Check Sphere on Plane ==
  x : Inport
  y : Inport  Port=2
  Abs : Abs  ZeroCross=off
  Abs1 : Abs  ZeroCross=off
  Check loc x-axis : simulink/Logic and Bit Operations/Compare To Constant  relop=<  const=plane_lenx  OutDataTypeStr=boolean  ZeroCross=off
  Check loc y-axis : simulink/Logic and Bit Operations/Compare To Constant  relop=<  const=plane_leny  OutDataTypeStr=boolean  ZeroCross=off
  Data Type Conversion : DataTypeConversion
  Gain : Gain  Gain=2
  Gain1 : Gain  Gain=2
  Logical Operator : Logic  AllPortsSameDT=off  OutDataTypeStr=boolean
  En : Outport
  wires:
  Check loc y-axis/1 -> Logical Operator/2
  Abs1/1 -> Check loc y-axis/1
  Abs/1 -> Check loc x-axis/1
  Gain1/1 -> Abs1/1
  Gain/1 -> Abs/1
  x/1 -> Gain/1
  Data Type Conversion/1 -> En/1
  y/1 -> Gain1/1
  Logical Operator/1 -> Data Type Conversion/1
  Check loc x-axis/1 -> Logical Operator/1

== system simulationBallCatching/Plant/Basket/Contact1/Demux ==
  Frc : Inport
  Demux : Demux
  Simulink-PS Converter{,1..2,6} (4 alike) : nesl_utility/Simulink-PS Converter  PhysicalDomain=network_engine_domain  SubClassName=ps_input  LeftPortType=input  RightPortType=output  PseudoPeriodic=off  Frequencies=[]  NoiseDistribution=none  NoiseParameters=[]  Unit=1  AffineConversion=off  FilteringAndDerivatives=zero  SimscapeFilterOrder=1  InputFilterTimeConstant=0.001  UdotUserProvided=1
  FSph : PMIOPort  Port=1  Side=Right
  TSph : PMIOPort  Port=2  Side=Right
  FPla : PMIOPort  Port=3  Side=Right
  TPla : PMIOPort  Port=4  Side=Right
  wires:
  Frc/1 -> Demux/1
  Demux/1 -> Simulink-PS Converter/1
  Demux/2 -> Simulink-PS Converter1/1
  Demux/4 -> Simulink-PS Converter2/1
  Demux/3 -> Simulink-PS Converter6/1
  connections:
  Simulink-PS Converter2/RConn1 -- TPla/RConn1
  Simulink-PS Converter/RConn1 -- FSph/RConn1
  Simulink-PS Converter1/RConn1 -- TSph/RConn1
  Simulink-PS Converter6/RConn1 -- FPla/RConn1

== system simulationBallCatching/Plant/Basket/Contact1/Enable Outputs ==
  Frc : Inport
  En : Inport  Port=2
  FrameSep : Inport  Port=3
  Bus Creator1 : BusCreator  Inputs=7
  Bus Selector : BusSelector  OutputSignals=Normal Force,Friction Force,Penetration,Penetration Vel,Spr Force,Damp Force
  Demux : Demux  Outputs=[1 3 1 1 1 1]
  Mux : Mux  Inputs=6
  Product : Product
  Out : Outport
  wires:
  Demux/2 -> Bus Creator1/2  "Friction Force"
  Demux/1 -> Bus Creator1/1  "Normal Force"
  Demux/6 -> Bus Creator1/6  "Damp Force"
  Demux/4 -> Bus Creator1/4  "Penetration Vel"
  Demux/5 -> Bus Creator1/5  "Spr Force"
  Demux/3 -> Bus Creator1/3  "Penetration"
  Product/1 -> Demux/1
  En/1 -> Product/1
  Mux/1 -> Product/2
  Bus Selector/3 -> Mux/3  "<Penetration>"
  Bus Creator1/1 -> Out/1
  Bus Selector/2 -> Mux/2  "<Friction Force>"
  Frc/1 -> Bus Selector/1
  Bus Selector/4 -> Mux/4  "<Penetration Vel>"
  FrameSep/1 -> Bus Creator1/7
  Bus Selector/1 -> Mux/1  "<Normal Force>"
  Bus Selector/6 -> Mux/6  "<Damp Force>"
  Bus Selector/5 -> Mux/5  "<Spr Force>"

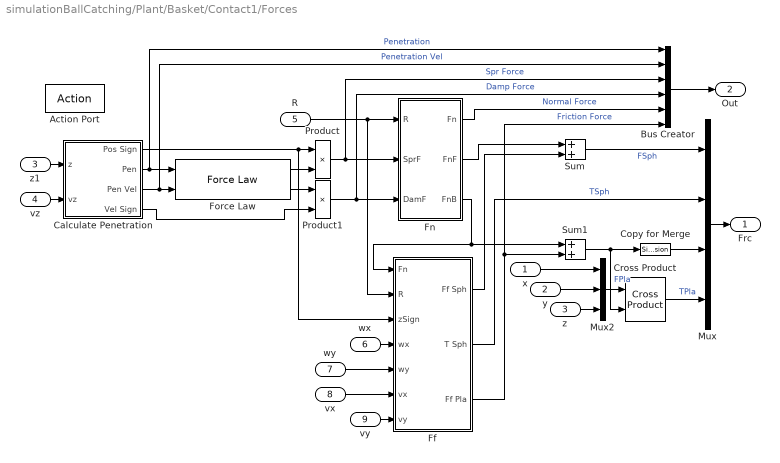
== system simulationBallCatching/Plant/Basket/Contact1/Forces ==
  x : Inport
  y : Inport  Port=2
  z : Inport  Port=3
  vz : Inport  Port=4
  R : Inport  Port=5
  wx : Inport  Port=6
  wy : Inport  Port=7
  vx : Inport  Port=8
  vy : Inport  Port=9
  Action Port : ActionPort  ActionType=then
  Bus Creator : BusCreator  Inputs=6
  Calculate Penetration : Subsystem
  Copy for Merge : SignalConversion  OverrideOpt=off
  Cross Product : Contact_Forces_Lib/Math/Cross Product
      settings: SourceProductName=Simscape Multibody Contact Forces Library
  Ff : Subsystem
  Fn : Subsystem
  Force Law : Contact_Forces_Lib/Force Law  OverrideUsingVariant=Linear
      settings: SourceProductName=Simscape Multibody Contact Forces Library
  Mux : Mux
  Mux2 : Mux  Inputs=3
  Product : Product
  Product1 : Product
  Sum : Sum
  Sum1 : Sum
  z1 : InportShadow  Port=3
  Frc : Outport
  Out : Outport  Port=2
  wires:
  Copy for Merge/1 -> Mux/3
  vx/1 -> Ff/6(vx)
  Product1/1 -> Bus Creator/4, Fn/3(DamF)  "Damp Force"
  Product/1 -> Bus Creator/3, Fn/2(SprF)  "Spr Force"
  Fn/2(FnF) -> Sum/1
  Mux/1 -> Frc/1
  Bus Creator/1 -> Out/1
  Force Law/1 -> Product/2
  vz/1 -> Calculate Penetration/2(vz)
  z1/1 -> Calculate Penetration/1(z)
  Calculate Penetration/2(Pen) -> Bus Creator/1, Force Law/1  "Penetration"
  Calculate Penetration/3(Pen Vel) -> Bus Creator/2, Force Law/2  "Penetration Vel"
  Fn/3(FnB) -> Sum1/1, Ff/1(Fn)
  Calculate Penetration/1(Pos Sign) -> Ff/3(zSign), Product/1
  Calculate Penetration/4(Vel Sign) -> Product1/2
  R/1 -> Fn/1(R), Ff/2(R)
  Force Law/2 -> Product1/1
  Sum1/1 -> Copy for Merge/1, Cross Product/2  "FPla"
  Mux2/1 -> Cross Product/1
  Ff/1(Ff Sph) -> Sum/2
  Fn/1(Fn) -> Bus Creator/5  "Normal Force"
  y/1 -> Mux2/2
  z/1 -> Mux2/3
  x/1 -> Mux2/1
  Ff/3(Ff Pla) -> Sum1/2, Bus Creator/6  "Friction Force"
  vy/1 -> Ff/7(vy)
  wy/1 -> Ff/5(wy)
  wx/1 -> Ff/4(wx)
  Sum/1 -> Mux/1  "FSph"
  Ff/2(T Sph) -> Mux/2  "TSph"
  Cross Product/1 -> Mux/4  "TPla"

== system simulationBallCatching/Plant/Basket/Contact1/No Force ==
  Action Port : ActionPort  ActionType=else
  Zeros : Constant  Value=[0 0 0 0 0 0 0 0 0 0 0 0]  SampleTime=0
  Frc : Outport  InitialOutput=[0 0 0 0 0 0 0 0 0 0 0 0]
  wires:
  Zeros/1 -> Frc/1

== system simulationBallCatching/Plant/Basket/Contact1/Sensing ==
  PS-Simulink Converter{,1..8} (9 alike) : nesl_utility/PS-Simulink Converter  PhysicalDomain=network_engine_domain  SubClassName=ps_output  LeftPortType=input  RightPortType=output  PseudoPeriodic=off  Frequencies=[]  Unit=1  AffineConversion=off
  Transform Sensor : sm_lib/Frames and Transforms/Transform Sensor  MeasurementFrame=Base  SenseAngle=off  SenseAxis=off  SenseAngle1=off  SenseAngle2=off  SenseAngle3=off  SenseQ=off  SenseR=on  SenseOmegaX=on  SenseOmegaY=on  SenseOmegaZ=off  SenseOmega1=off  SenseOmega2=off  SenseOmega3=off  SenseQDot=off  SenseRDot=off  SenseAlphaX=off  SenseAlphaY=off  SenseAlphaZ=off  SenseAlpha1=off  SenseAlpha2=off  SenseAlpha3=off  SenseQDDot=off  SenseRDDot=off  SenseX=on  SenseY=on  SenseZ=on  SenseRad=off  SenseAzim=off  SenseDist=off  SenseInc=off  SenseXDot=on  SenseYDot=on  SenseZDot=on  SenseRadDot=off  SenseAzimDot=off  SenseDistDot=off  SenseIncDot=off  SenseXDDot=off  SenseYDDot=off  SenseZDDot=off  SenseRadDDot=off  SenseAzimDDot=off  SenseDistDDot=off  SenseIncDDot=off
  F : PMIOPort  Port=1  Side=Left
  B : PMIOPort  Port=2  Side=Left
  x : Outport
  y : Outport  Port=2
  z : Outport  Port=3
  vz : Outport  Port=4
  R : Outport  Port=5
  wx : Outport  Port=6
  wy : Outport  Port=7
  vx : Outport  Port=8
  vy : Outport  Port=9
  wires:
  PS-Simulink Converter1/1 -> vz/1
  PS-Simulink Converter/1 -> z/1
  PS-Simulink Converter2/1 -> R/1
  PS-Simulink Converter3/1 -> wx/1
  PS-Simulink Converter4/1 -> wy/1
  PS-Simulink Converter5/1 -> vx/1
  PS-Simulink Converter6/1 -> vy/1
  PS-Simulink Converter7/1 -> x/1
  PS-Simulink Converter8/1 -> y/1
  connections:
  Transform Sensor/RConn1 -- F/RConn1
  Transform Sensor/LConn1 -- B/RConn1
  Transform Sensor/RConn2 -- PS-Simulink Converter2/LConn1
  Transform Sensor/RConn3 -- PS-Simulink Converter3/LConn1
  PS-Simulink Converter4/LConn1 -- Transform Sensor/RConn4
  PS-Simulink Converter1/LConn1 -- Transform Sensor/RConn10
  Transform Sensor/RConn9 -- PS-Simulink Converter6/LConn1
  Transform Sensor/RConn8 -- PS-Simulink Converter5/LConn1
  Transform Sensor/RConn7 -- PS-Simulink Converter/LConn1
  PS-Simulink Converter7/LConn1 -- Transform Sensor/RConn5
  PS-Simulink Converter8/LConn1 -- Transform Sensor/RConn6

== system simulationBallCatching/Plant/Basket/Contact2/Check Sphere on Plane ==
  x : Inport
  y : Inport  Port=2
  Abs : Abs  ZeroCross=off
  Abs1 : Abs  ZeroCross=off
  Check loc x-axis : simulink/Logic and Bit Operations/Compare To Constant  relop=<  const=plane_lenx  OutDataTypeStr=boolean  ZeroCross=off
  Check loc y-axis : simulink/Logic and Bit Operations/Compare To Constant  relop=<  const=plane_leny  OutDataTypeStr=boolean  ZeroCross=off
  Data Type Conversion : DataTypeConversion
  Gain : Gain  Gain=2
  Gain1 : Gain  Gain=2
  Logical Operator : Logic  AllPortsSameDT=off  OutDataTypeStr=boolean
  En : Outport
  wires:
  Check loc y-axis/1 -> Logical Operator/2
  Abs1/1 -> Check loc y-axis/1
  Abs/1 -> Check loc x-axis/1
  Gain1/1 -> Abs1/1
  Gain/1 -> Abs/1
  x/1 -> Gain/1
  Data Type Conversion/1 -> En/1
  y/1 -> Gain1/1
  Logical Operator/1 -> Data Type Conversion/1
  Check loc x-axis/1 -> Logical Operator/1

== system simulationBallCatching/Plant/Basket/Contact2/Demux ==
  Frc : Inport
  Demux : Demux
  Simulink-PS Converter{,1..2,6} (4 alike) : nesl_utility/Simulink-PS Converter  PhysicalDomain=network_engine_domain  SubClassName=ps_input  LeftPortType=input  RightPortType=output  PseudoPeriodic=off  Frequencies=[]  NoiseDistribution=none  NoiseParameters=[]  Unit=1  AffineConversion=off  FilteringAndDerivatives=zero  SimscapeFilterOrder=1  InputFilterTimeConstant=0.001  UdotUserProvided=1
  FSph : PMIOPort  Port=1  Side=Right
  TSph : PMIOPort  Port=2  Side=Right
  FPla : PMIOPort  Port=3  Side=Right
  TPla : PMIOPort  Port=4  Side=Right
  wires:
  Frc/1 -> Demux/1
  Demux/1 -> Simulink-PS Converter/1
  Demux/2 -> Simulink-PS Converter1/1
  Demux/4 -> Simulink-PS Converter2/1
  Demux/3 -> Simulink-PS Converter6/1
  connections:
  Simulink-PS Converter2/RConn1 -- TPla/RConn1
  Simulink-PS Converter/RConn1 -- FSph/RConn1
  Simulink-PS Converter1/RConn1 -- TSph/RConn1
  Simulink-PS Converter6/RConn1 -- FPla/RConn1

== system simulationBallCatching/Plant/Basket/Contact2/Enable Outputs ==
  Frc : Inport
  En : Inport  Port=2
  FrameSep : Inport  Port=3
  Bus Creator1 : BusCreator  Inputs=7
  Bus Selector : BusSelector  OutputSignals=Normal Force,Friction Force,Penetration,Penetration Vel,Spr Force,Damp Force
  Demux : Demux  Outputs=[1 3 1 1 1 1]
  Mux : Mux  Inputs=6
  Product : Product
  Out : Outport
  wires:
  Demux/2 -> Bus Creator1/2  "Friction Force"
  Demux/1 -> Bus Creator1/1  "Normal Force"
  Demux/6 -> Bus Creator1/6  "Damp Force"
  Demux/4 -> Bus Creator1/4  "Penetration Vel"
  Demux/5 -> Bus Creator1/5  "Spr Force"
  Demux/3 -> Bus Creator1/3  "Penetration"
  Product/1 -> Demux/1
  En/1 -> Product/1
  Mux/1 -> Product/2
  Bus Selector/3 -> Mux/3  "<Penetration>"
  Bus Creator1/1 -> Out/1
  Bus Selector/2 -> Mux/2  "<Friction Force>"
  Frc/1 -> Bus Selector/1
  Bus Selector/4 -> Mux/4  "<Penetration Vel>"
  FrameSep/1 -> Bus Creator1/7
  Bus Selector/1 -> Mux/1  "<Normal Force>"
  Bus Selector/6 -> Mux/6  "<Damp Force>"
  Bus Selector/5 -> Mux/5  "<Spr Force>"

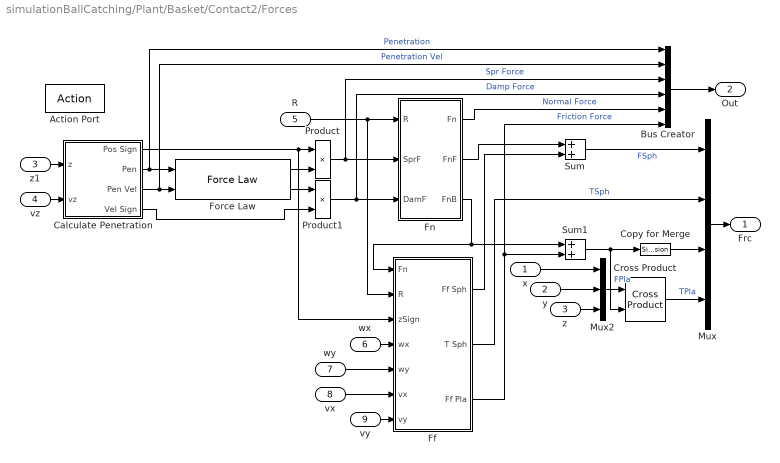
== system simulationBallCatching/Plant/Basket/Contact2/Forces ==
  x : Inport
  y : Inport  Port=2
  z : Inport  Port=3
  vz : Inport  Port=4
  R : Inport  Port=5
  wx : Inport  Port=6
  wy : Inport  Port=7
  vx : Inport  Port=8
  vy : Inport  Port=9
  Action Port : ActionPort  ActionType=then
  Bus Creator : BusCreator  Inputs=6
  Calculate Penetration : Subsystem
  Copy for Merge : SignalConversion  OverrideOpt=off
  Cross Product : Contact_Forces_Lib/Math/Cross Product
      settings: SourceProductName=Simscape Multibody Contact Forces Library
  Ff : Subsystem
  Fn : Subsystem
  Force Law : Contact_Forces_Lib/Force Law  OverrideUsingVariant=Linear
      settings: SourceProductName=Simscape Multibody Contact Forces Library
  Mux : Mux
  Mux2 : Mux  Inputs=3
  Product : Product
  Product1 : Product
  Sum : Sum
  Sum1 : Sum
  z1 : InportShadow  Port=3
  Frc : Outport
  Out : Outport  Port=2
  wires:
  Copy for Merge/1 -> Mux/3
  vx/1 -> Ff/6(vx)
  Product1/1 -> Bus Creator/4, Fn/3(DamF)  "Damp Force"
  Product/1 -> Bus Creator/3, Fn/2(SprF)  "Spr Force"
  Fn/2(FnF) -> Sum/1
  Mux/1 -> Frc/1
  Bus Creator/1 -> Out/1
  Force Law/1 -> Product/2
  vz/1 -> Calculate Penetration/2(vz)
  z1/1 -> Calculate Penetration/1(z)
  Calculate Penetration/2(Pen) -> Bus Creator/1, Force Law/1  "Penetration"
  Calculate Penetration/3(Pen Vel) -> Bus Creator/2, Force Law/2  "Penetration Vel"
  Fn/3(FnB) -> Sum1/1, Ff/1(Fn)
  Calculate Penetration/1(Pos Sign) -> Ff/3(zSign), Product/1
  Calculate Penetration/4(Vel Sign) -> Product1/2
  R/1 -> Fn/1(R), Ff/2(R)
  Force Law/2 -> Product1/1
  Sum1/1 -> Copy for Merge/1, Cross Product/2  "FPla"
  Mux2/1 -> Cross Product/1
  Ff/1(Ff Sph) -> Sum/2
  Fn/1(Fn) -> Bus Creator/5  "Normal Force"
  y/1 -> Mux2/2
  z/1 -> Mux2/3
  x/1 -> Mux2/1
  Ff/3(Ff Pla) -> Sum1/2, Bus Creator/6  "Friction Force"
  vy/1 -> Ff/7(vy)
  wy/1 -> Ff/5(wy)
  wx/1 -> Ff/4(wx)
  Sum/1 -> Mux/1  "FSph"
  Ff/2(T Sph) -> Mux/2  "TSph"
  Cross Product/1 -> Mux/4  "TPla"

== system simulationBallCatching/Plant/Basket/Contact2/No Force ==
  Action Port : ActionPort  ActionType=else
  Zeros : Constant  Value=[0 0 0 0 0 0 0 0 0 0 0 0]  SampleTime=0
  Frc : Outport  InitialOutput=[0 0 0 0 0 0 0 0 0 0 0 0]
  wires:
  Zeros/1 -> Frc/1

== system simulationBallCatching/Plant/Basket/Contact2/Sensing ==
  PS-Simulink Converter{,1..8} (9 alike) : nesl_utility/PS-Simulink Converter  PhysicalDomain=network_engine_domain  SubClassName=ps_output  LeftPortType=input  RightPortType=output  PseudoPeriodic=off  Frequencies=[]  Unit=1  AffineConversion=off
  Transform Sensor : sm_lib/Frames and Transforms/Transform Sensor  MeasurementFrame=Base  SenseAngle=off  SenseAxis=off  SenseAngle1=off  SenseAngle2=off  SenseAngle3=off  SenseQ=off  SenseR=on  SenseOmegaX=on  SenseOmegaY=on  SenseOmegaZ=off  SenseOmega1=off  SenseOmega2=off  SenseOmega3=off  SenseQDot=off  SenseRDot=off  SenseAlphaX=off  SenseAlphaY=off  SenseAlphaZ=off  SenseAlpha1=off  SenseAlpha2=off  SenseAlpha3=off  SenseQDDot=off  SenseRDDot=off  SenseX=on  SenseY=on  SenseZ=on  SenseRad=off  SenseAzim=off  SenseDist=off  SenseInc=off  SenseXDot=on  SenseYDot=on  SenseZDot=on  SenseRadDot=off  SenseAzimDot=off  SenseDistDot=off  SenseIncDot=off  SenseXDDot=off  SenseYDDot=off  SenseZDDot=off  SenseRadDDot=off  SenseAzimDDot=off  SenseDistDDot=off  SenseIncDDot=off
  F : PMIOPort  Port=1  Side=Left
  B : PMIOPort  Port=2  Side=Left
  x : Outport
  y : Outport  Port=2
  z : Outport  Port=3
  vz : Outport  Port=4
  R : Outport  Port=5
  wx : Outport  Port=6
  wy : Outport  Port=7
  vx : Outport  Port=8
  vy : Outport  Port=9
  wires:
  PS-Simulink Converter1/1 -> vz/1
  PS-Simulink Converter/1 -> z/1
  PS-Simulink Converter2/1 -> R/1
  PS-Simulink Converter3/1 -> wx/1
  PS-Simulink Converter4/1 -> wy/1
  PS-Simulink Converter5/1 -> vx/1
  PS-Simulink Converter6/1 -> vy/1
  PS-Simulink Converter7/1 -> x/1
  PS-Simulink Converter8/1 -> y/1
  connections:
  Transform Sensor/RConn1 -- F/RConn1
  Transform Sensor/LConn1 -- B/RConn1
  Transform Sensor/RConn2 -- PS-Simulink Converter2/LConn1
  Transform Sensor/RConn3 -- PS-Simulink Converter3/LConn1
  PS-Simulink Converter4/LConn1 -- Transform Sensor/RConn4
  PS-Simulink Converter1/LConn1 -- Transform Sensor/RConn10
  Transform Sensor/RConn9 -- PS-Simulink Converter6/LConn1
  Transform Sensor/RConn8 -- PS-Simulink Converter5/LConn1
  Transform Sensor/RConn7 -- PS-Simulink Converter/LConn1
  PS-Simulink Converter7/LConn1 -- Transform Sensor/RConn5
  PS-Simulink Converter8/LConn1 -- Transform Sensor/RConn6

== system simulationBallCatching/Plant/Basket/Contact3/Check Sphere on Plane ==
  x : Inport
  y : Inport  Port=2
  Abs : Abs  ZeroCross=off
  Abs1 : Abs  ZeroCross=off
  Check loc x-axis : simulink/Logic and Bit Operations/Compare To Constant  relop=<  const=plane_lenx  OutDataTypeStr=boolean  ZeroCross=off
  Check loc y-axis : simulink/Logic and Bit Operations/Compare To Constant  relop=<  const=plane_leny  OutDataTypeStr=boolean  ZeroCross=off
  Data Type Conversion : DataTypeConversion
  Gain : Gain  Gain=2
  Gain1 : Gain  Gain=2
  Logical Operator : Logic  AllPortsSameDT=off  OutDataTypeStr=boolean
  En : Outport
  wires:
  Check loc y-axis/1 -> Logical Operator/2
  Abs1/1 -> Check loc y-axis/1
  Abs/1 -> Check loc x-axis/1
  Gain1/1 -> Abs1/1
  Gain/1 -> Abs/1
  x/1 -> Gain/1
  Data Type Conversion/1 -> En/1
  y/1 -> Gain1/1
  Logical Operator/1 -> Data Type Conversion/1
  Check loc x-axis/1 -> Logical Operator/1

== system simulationBallCatching/Plant/Basket/Contact3/Demux ==
  Frc : Inport
  Demux : Demux
  Simulink-PS Converter{,1..2,6} (4 alike) : nesl_utility/Simulink-PS Converter  PhysicalDomain=network_engine_domain  SubClassName=ps_input  LeftPortType=input  RightPortType=output  PseudoPeriodic=off  Frequencies=[]  NoiseDistribution=none  NoiseParameters=[]  Unit=1  AffineConversion=off  FilteringAndDerivatives=zero  SimscapeFilterOrder=1  InputFilterTimeConstant=0.001  UdotUserProvided=1
  FSph : PMIOPort  Port=1  Side=Right
  TSph : PMIOPort  Port=2  Side=Right
  FPla : PMIOPort  Port=3  Side=Right
  TPla : PMIOPort  Port=4  Side=Right
  wires:
  Frc/1 -> Demux/1
  Demux/1 -> Simulink-PS Converter/1
  Demux/2 -> Simulink-PS Converter1/1
  Demux/4 -> Simulink-PS Converter2/1
  Demux/3 -> Simulink-PS Converter6/1
  connections:
  Simulink-PS Converter2/RConn1 -- TPla/RConn1
  Simulink-PS Converter/RConn1 -- FSph/RConn1
  Simulink-PS Converter1/RConn1 -- TSph/RConn1
  Simulink-PS Converter6/RConn1 -- FPla/RConn1
